simulink model "Demonstration"  (R2012b)
settings: Solver=ode45  StartTime=0.0  StopTime=10.0  RelTol=1e-3
StartFcn:
  | openscopes
StopFcn:
  | openscopes
libraries: dspsrcs4 x2, fuzblock x1
settings Model: Creator=asus  LastModifiedBy=asus

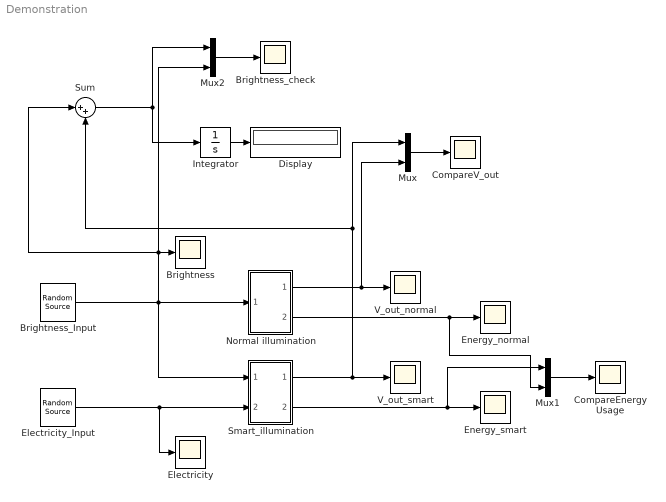
== system Demonstration ==
  Brightness : Scope
      settings: ShowLegends=on  YMin=-1  YMax=1  SaveName=ScopeData2
  Brightness_Input : dspsrcs4/Random Source  SrcType=Uniform  NormMethod=Ziggurat  CltLength=12  MinVal=0  MaxVal=1  MeanVal=0  VarVal=1  RepMode=Not repeatable  rawSeed=1  IsInherit=off  SampMode=Continuous  SampTime=1  SampFrame=1  DataType=Double  OutComplex=Real
  Brightness_check : Scope
      settings: ShowLegends=on  YMin=-1  YMax=1  SaveName=ScopeData8
  CompareEnergy Usage : Scope
      settings: ShowLegends=on  YMin=-1  YMax=1  SaveName=ScopeData9
  CompareV_out : Scope
      settings: ShowLegends=on  YMin=-1  YMax=1  SaveName=ScopeData6
  Display : Display
  Electricity : Scope
      settings: ShowLegends=on  YMin=-1  YMax=1
  Electricity_Input : dspsrcs4/Random Source  SrcType=Uniform  NormMethod=Ziggurat  CltLength=12  MinVal=0  MaxVal=1  MeanVal=0  VarVal=1  RepMode=Not repeatable  rawSeed=1  IsInherit=off  SampMode=Continuous  SampTime=1  SampFrame=1  DataType=Double  OutComplex=Real
  Energy_normal : Scope
      settings: ShowLegends=on  YMin=2.77556e-17  YMax=0.9  SaveName=ScopeData5
  "Energy_smart " : Scope
      settings: ShowLegends=on  SaveName=ScopeData3
  Integrator : Integrator
  Mux : Mux  Inputs=2
  Mux1 : Mux  Inputs=2
  Mux2 : Mux  Inputs=2
  Normal illumination : Subsystem
  Smart_illumination : Subsystem
  Sum : Sum  Inputs=|++
  V_out_normal : Scope
      settings: ShowLegends=on  YMin=2.77556e-17  YMax=0.9  SaveName=ScopeData4
  V_out_smart : Scope
      settings: ShowLegends=on  YMin=2.77556e-17  YMax=0.9
  wires:
  Mux1/1 -> CompareEnergy Usage/1
  Mux/1 -> CompareV_out/1
  Sum/1 -> Integrator/1, Mux2/1
  Mux2/1 -> Brightness_check/1
  Integrator/1 -> Display/1
  Brightness_Input/1 -> Sum/1, Mux2/2, Brightness/1, Smart_illumination/1(In1), Normal illumination/1(Brightness)
  Electricity_Input/1 -> Smart_illumination/2(In2), Electricity/1
  Smart_illumination/2(Energy) -> "Energy_smart "/1, Mux1/1
  Normal illumination/2(Energy_normal) -> Energy_normal/1, Mux1/2
  Normal illumination/1(V_out) -> V_out_normal/1, Mux/2
  Smart_illumination/1(V_out) -> V_out_smart/1, Sum/2, Mux/1

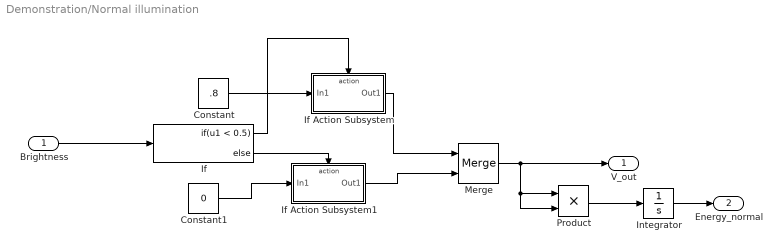
== system Demonstration/Normal illumination ==
  Brightness : Inport
  Constant : Constant  Value=.8
  Constant1 : Constant  Value=0
  If : If  IfExpression=u1 < 0.5
  If Action Subsystem : Subsystem  TreatAsAtomicUnit=on
  If Action Subsystem1 : Subsystem  TreatAsAtomicUnit=on
  Integrator : Integrator
  Merge : Merge
  Product : Product  RndMeth=Zero
  V_out : Outport
  Energy_normal : Outport  Port=2
  wires:
  If Action Subsystem/1(Out1) -> Merge/1
  Brightness/1 -> If/1
  Constant1/1 -> If Action Subsystem1/1(In1)
  If/2 -> If Action Subsystem1/Action
  Product/1 -> Integrator/1
  Merge/1 -> V_out/1, Product/2, Product/1
  If Action Subsystem1/1(Out1) -> Merge/2
  Integrator/1 -> Energy_normal/1
  If/1 -> If Action Subsystem/Action
  Constant/1 -> If Action Subsystem/1(In1)

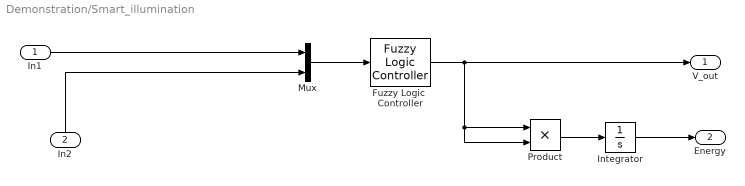
== system Demonstration/Smart_illumination ==
  In1 : Inport
  In2 : Inport  Port=2
  Fuzzy Logic  Controller : fuzblock/Fuzzy Logic  Controller  fis=smart_illumination
      link override FIS Wizard/AggMethod1: Function=max  Inputs=9
  Integrator : Integrator
  Mux : Mux  Inputs=2
  Product : Product  RndMeth=Zero
  V_out : Outport
  Energy : Outport  Port=2
  wires:
  Product/1 -> Integrator/1
  Integrator/1 -> Energy/1
  In1/1 -> Mux/1
  In2/1 -> Mux/2
  Fuzzy Logic  Controller/1 -> V_out/1, Product/1, Product/2
  Mux/1 -> Fuzzy Logic  Controller/1

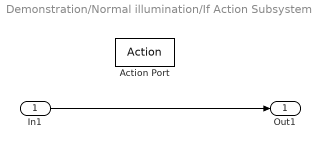
== system Demonstration/Normal illumination/If Action Subsystem ==
  In1 : Inport
  Action Port : ActionPort  ActionType=then
  Out1 : Outport
  wires:
  In1/1 -> Out1/1

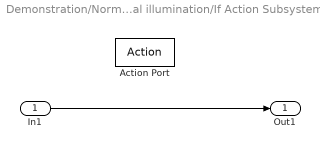
== system Demonstration/Normal illumination/If Action Subsystem1 ==
  In1 : Inport
  Action Port : ActionPort  ActionType=else
  Out1 : Outport
  wires:
  In1/1 -> Out1/1
